simulink model "basicModel"  (R2017b)
settings: Solver=ode3  StartTime=0.0  StopTime=30  FixedStep=0.01  RelTol=1e-3  EnableMultiTasking=on
InitFcn:
  | clear;
  | clc;
  | Iniparameters
StopFcn:
  | simplot
values from neighbouring files (symbols this model uses):
  aaa = inv([kf kf kf kf ... (first row only)    [copterpara.m]
  g = 9.8    [copterpara.m]
  Ixx = 19.688e-3    (= 0.019688)    [copterpara.m]
  Iyy = 19.688e-3    (= 0.019688)    [copterpara.m]
  Izz = 3.938e-2    (= 0.03938)    [copterpara.m]
  kdphi = 8    [controlpara.m]
  kdpsai = 40    [controlpara.m]
  kdtheta = kdphi    (= 8)    [controlpara.m]
  kdx = 0.55    [controlpara.m]
  kdy = 2.0    (= 2)    [controlpara.m]
  kdz = 2.4    [controlpara.m]
  kf = 3.13e-5    (= 3.13e-05)    [copterpara.m]
  kipsai = 10    [controlpara.m]
  Kis = 0.00    (= 0)    [Iniparameters.m]
  kix = 0.001    [controlpara.m]
  kiy = 0.001    [controlpara.m]
  kiz = 0.001    [controlpara.m]
  km = 7.5e-7    (= 7.5e-07)    [copterpara.m]
  kpphi = 25    [controlpara.m]
  kppsai = 20    [controlpara.m]
  Kps = 20    [Iniparameters.m]
  kptheta = kpphi    (= 25)    [controlpara.m]
  kpx = 0.75    [controlpara.m]
  kpy = 1.4    [controlpara.m]
  kpz = 2.9    [controlpara.m]
  L = 0.25    [copterpara.m]
  m = 0.75    [copterpara.m]
  xf = 0    [controlpara.m]
  yaw = 0    [copterpara.m]
  yf = 0    [controlpara.m]
  zf = 5    [controlpara.m]
libraries: aerolibconvert2 x19, aerolibutil x7, sharedtransform x3, dspfdesign x1, sharedutil x1, aerolibnav x1
settings Model: Creator=KingBoy  LastModifiedBy=KingBoy
settings DataIOCC: LimitDataPoints=on  SaveFormat=Array
settings OptimizationCC: LifeSpan=inf
settings DebuggingCC: UnderspecifiedInitializationDetection=Classic  MergeDetectMultiDrivingBlocksExec=none  SolverPrmCheckMsg=warning  AllowSymbolicDim=off  SFUnexpectedBacktrackingDiag=warning  SFNoUnconditionalDefaultTransitionDiag=warning  SFExecutionAtInitializationDiag=none
settings HardwareCC: ProdBitPerPointer=32  ProdBitPerSizeT=32  ProdBitPerPtrDiffT=32  ProdLargestAtomicFloat=None  ProdIntDivRoundTo=Undefined  ProdEndianess=Unspecified  ProdWordSize=32  ProdHWDeviceType=32-bit Generic
settings ModelReferenceCC: PropagateSignalLabelsOutOfModel=off
settings CodeAppCC: StateflowObjectComments=on
settings GRTTargetCC: TargetLangStandard=C89/C90 (ANSI)  GeneratePreprocessorConditionals=Disable all
settings ConfigComp: CovMetricSettings=dw  CovHtmlReporting=on  CovSaveCumulativeToWorkspaceVar=on  CovSaveSingleToWorkspaceVar=on  CovExternalEMLEnable=off  CovSFcnEnable=off

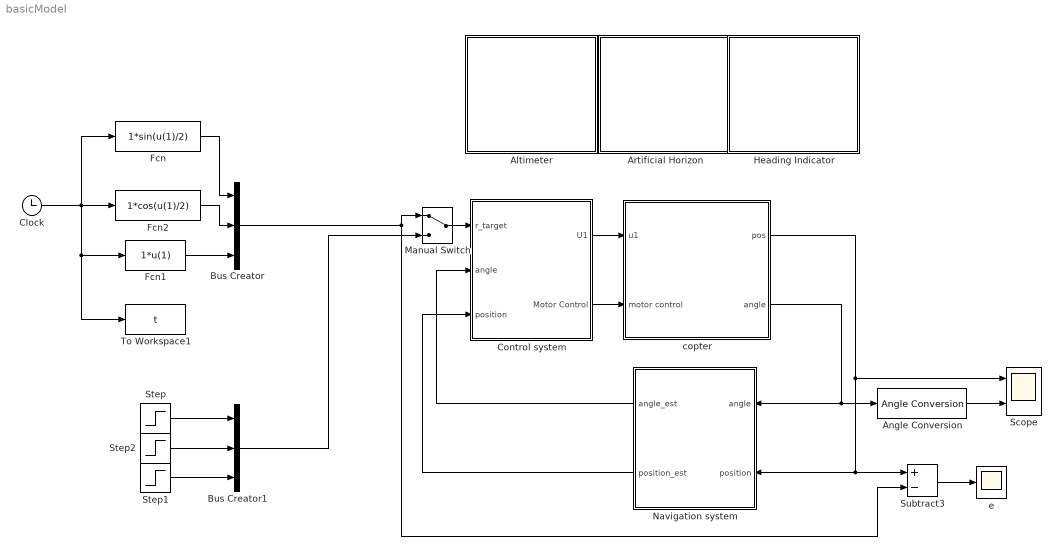
== system basicModel ==
  Altimeter : Subsystem  DialogController=aeroblksHMICreateDDGDialog  IsWebBlock=on  mask(MWDashboardBlock){webBlockId=0f36f96d-2aae-4714-b8ea-94d9972957ff, webBlockType=altimeter, ShowInLibBrowser=on, ShowInitialText=on, HMISrcModelName=basicModel}
      mask prompts: webBlockId "WebBlock Id"; webBlockType "WebBlock Type"; HMISrcModelName "Source Model"
      mask help: aeroblksHMI:aeroblkhmi:AltimeterDialogDesc
      mask Help: eval('asbhmihelp(''altimeter'')');
      mask Display:
      | if strcmp(get_param(bdroot(gcb),'BlockDiagramType'), 'library')
      |  image([(matlabroot) '/toolbox/aeroblks/aeroblks/hmi/icons/AltimeterIcon.svg'])
      | end
  Angle Conversion : aerolibconvert2/Angle Conversion  IU=rad  OU=deg
  Artificial Horizon : Subsystem  DialogController=aeroblksHMICreateDDGDialog  IsWebBlock=on  mask(MWDashboardBlock){webBlockId=fe52ae29-8116-408a-bf44-916d05edf52b, webBlockType=artificialhorizon, ShowInLibBrowser=on, ShowInitialText=on, HMISrcModelName=basicModel}
      mask prompts: webBlockId "WebBlock Id"; webBlockType "WebBlock Type"; HMISrcModelName "Source Model"
      mask help: aeroblksHMI:aeroblkhmi:ArtificialHorizonDialogDesc
      mask Help: eval('asbhmihelp(''artificialhorizon'')');
      mask Display:
      | if strcmp(get_param(bdroot(gcb),'BlockDiagramType'), 'library')
      |  image([(matlabroot) '/toolbox/aeroblks/aeroblks/hmi/icons/ArtificialHorizonIcon.svg'])
      | end
  Bus Creator : BusCreator  Inputs=3
  Bus Creator1 : BusCreator  Inputs=3
  Clock : Clock
  Control system : Subsystem
  Fcn : Fcn  Expr=1*sin(u(1)/2)
  Fcn1 : Fcn  Expr=1*u(1)
  Fcn2 : Fcn  Expr=1*cos(u(1)/2)
  Heading Indicator : Subsystem  DialogController=aeroblksHMICreateDDGDialog  IsWebBlock=on  mask(MWDashboardBlock){webBlockId=cbbc731a-5116-4125-a70b-a05ae3f6ae8f, webBlockType=headingindicator, ShowInLibBrowser=on, ShowInitialText=on, HMISrcModelName=basicModel}
      mask prompts: webBlockId "WebBlock Id"; webBlockType "WebBlock Type"; HMISrcModelName "Source Model"
      mask help: aeroblksHMI:aeroblkhmi:HeadingIndicatorDialogDesc
      mask Help: eval('asbhmihelp(''headingindicator'')');
      mask Display:
      | if strcmp(get_param(bdroot(gcb),'BlockDiagramType'), 'library')
      |  image([(matlabroot) '/toolbox/aeroblks/aeroblks/hmi/icons/HeadingIndicatorIcon.svg'])
      | end
  Manual Switch : ManualSwitch
  Navigation system : Subsystem
  Scope : Scope  NumInputPorts=2
  Step : Step  Time=0  After=xf  SampleTime=0
  Step1 : Step  Time=0  After=zf  SampleTime=0
  Step2 : Step  Time=0  After=yf  SampleTime=0
  Subtract3 : Sum  Inputs=+-
  To Workspace1 : ToWorkspace  VariableName=t  SampleTime=-1
      settings: Save2DSignal=2-D array (concatenate along first dimension)
  copter : Subsystem
  e : Scope
  wires:
  Angle Conversion/1 -> Scope/2
  Clock/1 -> To Workspace1/1, Fcn1/1, Fcn/1, Fcn2/1
  Fcn/1 -> Bus Creator/1
  Fcn2/1 -> Bus Creator/2
  Fcn1/1 -> Bus Creator/3
  Subtract3/1 -> e/1
  Bus Creator/1 -> Manual Switch/1, Subtract3/2
  copter/2(angle) -> Angle Conversion/1, Navigation system/1(angle)
  copter/1(pos) -> Scope/1, Subtract3/1, Navigation system/2(position)
  Control system/1(U1) -> copter/1(u1)
  Control system/2(Motor Control) -> copter/2(motor control)
  Navigation system/1(angle_est) -> Control system/2(angle)
  Navigation system/2(position_est) -> Control system/3(position)
  Manual Switch/1 -> Control system/1(r_target)
  Bus Creator1/1 -> Manual Switch/2
  Step/1 -> Bus Creator1/1
  Step1/1 -> Bus Creator1/3
  Step2/1 -> Bus Creator1/2

== system basicModel/Altimeter ==

== system basicModel/Artificial Horizon ==

== system basicModel/Control system ==
  r_target : Inport
  angle : Inport  Port=2
  position : Inport  Port=3
  Attitude Control : Subsystem
  PositionControl : Subsystem
  U1 : Outport
  Motor Control : Outport  Port=2
  wires:
  PositionControl/2(angle_des) -> Attitude Control/1(angle_des)
  angle/1 -> Attitude Control/2(angle_est)
  PositionControl/1(u1) -> U1/1
  Attitude Control/1(motor control) -> Motor Control/1
  position/1 -> PositionControl/2(r_pos)
  r_target/1 -> PositionControl/1(r_target)

== system basicModel/Heading Indicator ==

== system basicModel/Navigation system ==
  angle : Inport
  position : Inport  Port=2
  Attitude estimate : Subsystem
  gps sensor : Subsystem
  inertial sensor : Subsystem
  position estimate : Subsystem
  angle_est : Outport
  position_est : Outport  Port=2
  wires:
  position/1 -> gps sensor/1(pos)
  angle/1 -> inertial sensor/1(angle)
  gps sensor/1(GPSpos) -> position estimate/1(GPSpos)
  position estimate/1(postion_est) -> position_est/1
  inertial sensor/1(acc gyro mag) -> Attitude estimate/1(acc gyro mag)
  Attitude estimate/1(angle_est) -> angle_est/1
  inertial sensor/2(acc gyro mag1) -> Attitude estimate/2(acc gyro mag1)

== system basicModel/copter ==
  u1 : Inport
  motor control : Inport  Port=2
  Moter Dynamic : Subsystem
  Rigid Body Dynamic : Subsystem
  pos : Outport
  angle : Outport  Port=2
  wires:
  u1/1 -> Moter Dynamic/1(u1)
  Rigid Body Dynamic/2(angle) -> angle/1
  motor control/1 -> Moter Dynamic/2(d_wphi)
  Rigid Body Dynamic/1(xyzt) -> pos/1
  Moter Dynamic/2(M) -> Rigid Body Dynamic/2(M)
  Moter Dynamic/1(T) -> Rigid Body Dynamic/1(T)

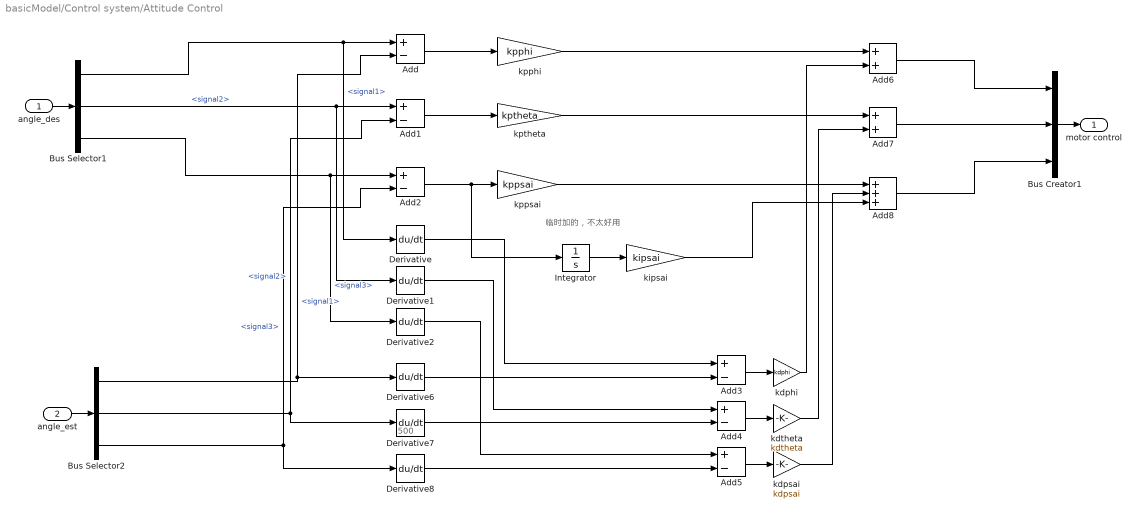
== system basicModel/Control system/Attitude Control ==
  note: 临时加的，不太好用
  note: 500
  angle_des : Inport
  angle_est : Inport  Port=2
  Add{,1..5} (6 alike) : Sum  Inputs=+-
  Add6 : Sum
  Add7 : Sum
  Add8 : Sum  Inputs=+++
  Bus Creator1 : BusCreator  Inputs=3
  Bus Selector1 : BusSelector  OutputSignals=signal1,signal2,signal3
  Bus Selector2 : BusSelector  OutputSignals=signal1,signal2,signal3
  Derivative{,1..2,6..8} (6 alike) : Derivative  CoefficientInTFapproximation=500
  Integrator : Integrator
  kdphi : Gain  Gain=kdphi
  kdpsai : Gain  Gain=kdpsai
  kdtheta : Gain  Gain=kdtheta
  kipsai : Gain  Gain=kipsai
  kpphi : Gain  Gain=kpphi
  kppsai : Gain  Gain=kppsai
  kptheta : Gain  Gain=kptheta
  motor control : Outport
  wires:
  Bus Selector1/1 -> Add/1, Derivative/1  "<signal1>"
  Bus Selector2/1 -> Add/2, Derivative6/1  "<signal1>"
  Add/1 -> kpphi/1
  Bus Selector1/2 -> Derivative1/1, Add1/1  "<signal2>"
  Bus Selector2/2 -> Add1/2, Derivative7/1  "<signal2>"
  Add1/1 -> kptheta/1
  Add2/1 -> Integrator/1, kppsai/1
  Bus Selector1/3 -> Derivative2/1, Add2/1  "<signal3>"
  Bus Selector2/3 -> Add2/2, Derivative8/1  "<signal3>"
  Add3/1 -> kdphi/1
  Add4/1 -> kdtheta/1
  Add5/1 -> kdpsai/1
  kpphi/1 -> Add6/1
  kdphi/1 -> Add6/2
  kptheta/1 -> Add7/1
  kdtheta/1 -> Add7/2
  kppsai/1 -> Add8/1
  kdpsai/1 -> Add8/2
  Derivative/1 -> Add3/1
  Derivative1/1 -> Add4/1
  Derivative2/1 -> Add5/1
  Derivative6/1 -> Add3/2
  Derivative7/1 -> Add4/2
  Derivative8/1 -> Add5/2
  angle_est/1 -> Bus Selector2/1
  angle_des/1 -> Bus Selector1/1
  Bus Creator1/1 -> motor control/1
  Add6/1 -> Bus Creator1/1
  Add7/1 -> Bus Creator1/2
  Add8/1 -> Bus Creator1/3
  Integrator/1 -> kipsai/1
  kipsai/1 -> Add8/3

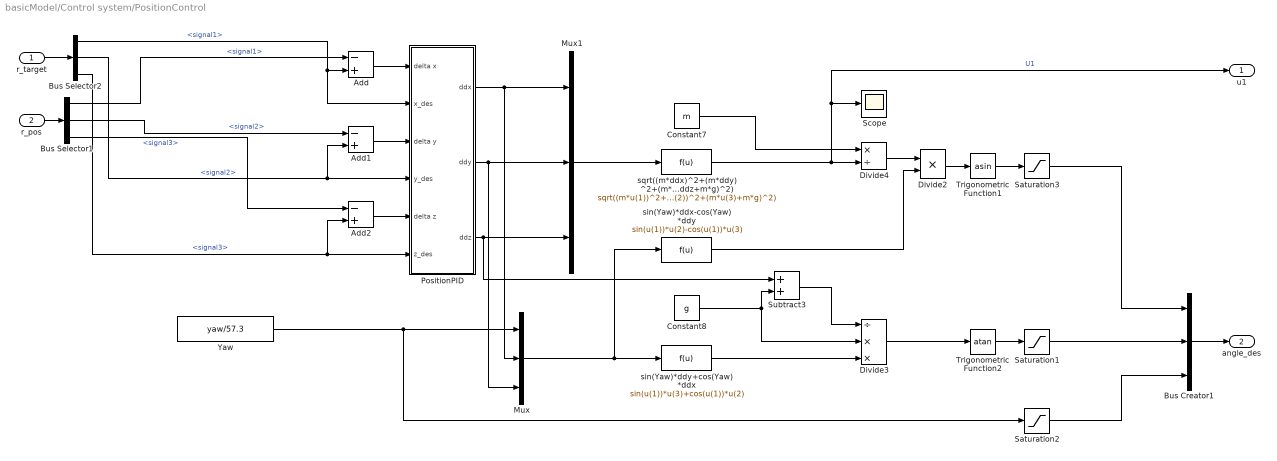
== system basicModel/Control system/PositionControl ==
  r_target : Inport
  r_pos : Inport  Port=2
  Add : Sum  Inputs=-+
  Add1 : Sum  Inputs=-+
  Add2 : Sum  Inputs=-+
  Bus Creator1 : BusCreator  Inputs=3
  Bus Selector1 : BusSelector  OutputSignals=signal1,signal2,signal3
  Bus Selector2 : BusSelector  OutputSignals=signal1,signal2,signal3
  Constant7 : Constant  Value=m
  Constant8 : Constant  Value=g
  Divide2 : Product  Inputs=**
  Divide3 : Product  Inputs=/**
  Divide4 : Product  Inputs=*/
  Mux : Mux  Inputs=3
  Mux1 : Mux  Inputs=3
  PositionPID : Subsystem
  Saturation1 : Saturate  UpperLimit=90/57.3  LowerLimit=-90/57.3
  Saturation2 : Saturate  UpperLimit=90/57.3  LowerLimit=-90/57.3
  Saturation3 : Saturate  UpperLimit=90/57.3  LowerLimit=-90/57.3
  Scope : Scope
  Subtract3 : Sum
  Trigonometric Function1 : Trigonometry  Operator=asin
  Trigonometric Function2 : Trigonometry  Operator=atan
  Yaw : Constant  Value=yaw/57.3
  sin(Yaw)*ddx-cos(Yaw)*ddy : Fcn  Expr=sin(u(1))*u(2)-cos(u(1))*u(3)
  sin(Yaw)*ddy+cos(Yaw)*ddx : Fcn  Expr=sin(u(1))*u(3)+cos(u(1))*u(2)
  sqrt((m*ddx)^2+(m*ddy)^2+(m*ddz+m*g)^2) : Fcn  Expr=sqrt((m*u(1))^2+(m*u(2))^2+(m*u(3)+m*g)^2)
  u1 : Outport
  angle_des : Outport  Port=2
  wires:
  Bus Selector1/1 -> Add/1  "<signal1>"
  Add/1 -> PositionPID/1(delta x)
  Bus Selector1/2 -> Add1/1  "<signal2>"
  Bus Selector2/2 -> Add1/2, PositionPID/4(y_des)  "<signal2>"
  Add1/1 -> PositionPID/3(delta y)
  Bus Selector1/3 -> Add2/1  "<signal3>"
  Bus Selector2/3 -> Add2/2, PositionPID/6(z_des)  "<signal3>"
  Add2/1 -> PositionPID/5(delta z)
  PositionPID/2(ddy) -> Mux/3, Mux1/2
  sqrt((m*ddx)^2+(m*ddy)^2+(m*ddz+m*g)^2)/1 -> u1/1, Scope/1, Divide4/2  "U1"
  PositionPID/3(ddz) -> Subtract3/1, Mux1/3
  sin(Yaw)*ddx-cos(Yaw)*ddy/1 -> Divide2/2
  Divide3/1 -> Trigonometric Function2/1
  Constant7/1 -> Divide4/1
  Divide4/1 -> Divide2/1
  Constant8/1 -> Divide3/2, Subtract3/2
  Trigonometric Function2/1 -> Saturation1/1
  Trigonometric Function1/1 -> Saturation3/1
  Divide2/1 -> Trigonometric Function1/1
  PositionPID/1(ddx) -> Mux1/1, Mux/2
  Yaw/1 -> Mux/1, Saturation2/1
  Subtract3/1 -> Divide3/1
  Saturation3/1 -> Bus Creator1/1
  Saturation1/1 -> Bus Creator1/2
  Saturation2/1 -> Bus Creator1/3
  Mux/1 -> sin(Yaw)*ddx-cos(Yaw)*ddy/1, sin(Yaw)*ddy+cos(Yaw)*ddx/1
  Mux1/1 -> sqrt((m*ddx)^2+(m*ddy)^2+(m*ddz+m*g)^2)/1
  sin(Yaw)*ddy+cos(Yaw)*ddx/1 -> Divide3/3
  r_pos/1 -> Bus Selector1/1
  r_target/1 -> Bus Selector2/1
  Bus Selector2/1 -> PositionPID/2(x_des), Add/2  "<signal1>"
  Bus Creator1/1 -> angle_des/1

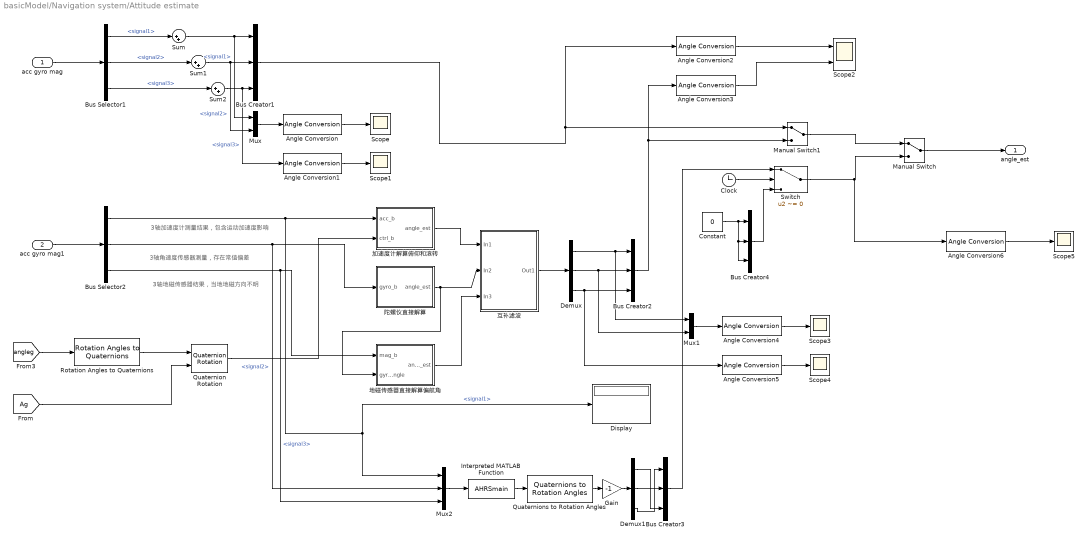
== system basicModel/Navigation system/Attitude estimate ==
  note: 3轴加速度计测量结果，包含运动加速度影响
  note: 3轴角速度传感器测量，存在常值偏差
  note: 3轴地磁传感器结果，当地地磁方向不明
  acc gyro mag : Inport
  acc gyro mag1 : Inport  Port=2
  Angle Conversion{,1..6} (7 alike) : aerolibconvert2/Angle Conversion  IU=rad  OU=deg
  Bus Creator{1..4} (4 alike) : BusCreator  Inputs=3
  Bus Selector1 : BusSelector  OutputSignals=signal1,signal2,signal3
  Bus Selector2 : BusSelector  OutputSignals=signal1,signal2,signal3
  Clock : Clock
  Constant : Constant  Value=0
  Demux : Demux  Outputs=3
  Demux1 : Demux  Outputs=3
  Display : Display
  Gain : Gain  Gain=-1
  Interpreted MATLAB Function : MATLABFcn  MATLABFcn=AHRSmain
  Manual Switch : ManualSwitch
  Manual Switch1 : ManualSwitch
  Mux : Mux  Inputs=2
  Mux1 : Mux  Inputs=2
  Mux2 : Mux  Inputs=3
  Quaternion Rotation : aerolibutil/Quaternion Rotation
  Quaternions to Rotation Angles : sharedtransform/Quaternions to Rotation Angles  rotationOrder=ZYX
      settings: SourceProductBaseCode=AE
  Rotation Angles to Quaternions : sharedtransform/Rotation Angles to Quaternions  rotationOrder=ZYX
      settings: SourceProductName=Aerospace Blockset  SourceProductBaseCode=AE
  Scope{,1,3..5} (5 alike) : Scope
  Scope2 : Scope  NumInputPorts=2
  Sum : Sum  Inputs=|++
  Sum1 : Sum  Inputs=|++
  Sum2 : Sum  Inputs=|++
  Switch : Switch  Criteria=u2 ~= 0
  互补滤波 : Subsystem
  加速度计解算俯仰和滚转 : Subsystem
  地磁传感器直接解算偏航角 : Subsystem
  陀螺仪直接解算 : Subsystem
  angle_est : Outport
  wires:
  acc gyro mag/1 -> Bus Selector1/1
  Bus Creator1/1 -> Manual Switch1/1, Angle Conversion2/1
  Bus Selector1/1 -> Sum/1  "<signal1>"
  Bus Selector1/2 -> Sum1/1  "<signal2>"
  Bus Selector1/3 -> Sum2/1  "<signal3>"
  Sum/1 -> Mux/1, Bus Creator1/1  "<signal1>"
  Sum1/1 -> Mux/2, Bus Creator1/2  "<signal2>"
  Sum2/1 -> Angle Conversion1/1, Bus Creator1/3  "<signal3>"
  Mux/1 -> Angle Conversion/1
  Angle Conversion/1 -> Scope/1
  Angle Conversion1/1 -> Scope1/1
  acc gyro mag1/1 -> Bus Selector2/1
  Bus Selector2/3 -> Mux2/3, 地磁传感器直接解算偏航角/1(mag_b)  "<signal3>"
  Bus Selector2/2 -> Mux2/2, 陀螺仪直接解算/1(gyro_b)  "<signal2>"
  Rotation Angles to Quaternions/1 -> Quaternion Rotation/1
  [angleg] -> Rotation Angles to Quaternions/1
  [Ag] -> Quaternion Rotation/2
  Bus Selector2/1 -> Display/1, Mux2/1, 加速度计解算俯仰和滚转/1(acc_b)  "<signal1>"
  Quaternion Rotation/1 -> 加速度计解算俯仰和滚转/2(ctrl_b)
  加速度计解算俯仰和滚转/1(angle_est) -> 互补滤波/1(In1)
  陀螺仪直接解算/1(angle_est) -> 地磁传感器直接解算偏航角/2(gyro angle), 互补滤波/2(In2)
  互补滤波/1(Out1) -> Demux/1
  Demux/1 -> Mux1/1, Bus Creator2/1
  Demux/2 -> Mux1/2, Bus Creator2/2
  地磁传感器直接解算偏航角/1(angle_est) -> 互补滤波/3(In3)
  Bus Creator2/1 -> Manual Switch1/2, Angle Conversion3/1
  Manual Switch/1 -> angle_est/1
  Angle Conversion2/1 -> Scope2/1
  Angle Conversion3/1 -> Scope2/2
  Demux/3 -> Angle Conversion5/1, Bus Creator2/3
  Angle Conversion4/1 -> Scope3/1
  Angle Conversion5/1 -> Scope4/1
  Mux1/1 -> Angle Conversion4/1
  Mux2/1 -> Interpreted MATLAB Function/1
  Interpreted MATLAB Function/1 -> Quaternions to Rotation Angles/1
  Quaternions to Rotation Angles/1 -> Gain/1
  Angle Conversion6/1 -> Scope5/1
  Demux1/1 -> Bus Creator3/3
  Demux1/2 -> Bus Creator3/2
  Demux1/3 -> Bus Creator3/1
  Bus Creator3/1 -> Switch/1
  Gain/1 -> Demux1/1
  Clock/1 -> Switch/2
  Switch/1 -> Angle Conversion6/1, Manual Switch/2
  Constant/1 -> Bus Creator4/3, Bus Creator4/2, Bus Creator4/1
  Bus Creator4/1 -> Switch/3
  Manual Switch1/1 -> Manual Switch/1

== system basicModel/Navigation system/gps sensor ==
  pos : Inport
  Bus Creator1 : BusCreator  Inputs=3
  Bus Selector1 : BusSelector  OutputSignals=signal1,signal2,signal3
  Manual Switch : ManualSwitch  CurrentSetting=0
  Random Number : RandomNumber  Variance=100  Seed=10  SampleTime=0.01
  Random Number1 : RandomNumber  Variance=100  Seed=11  SampleTime=0.01
  Random Number2 : RandomNumber  Variance=100  Seed=12  SampleTime=0.01
  Scope : Scope
  Sum : Sum  Inputs=|++
  Sum1 : Sum  Inputs=|++
  Sum2 : Sum  Inputs=|++
  GPSpos : Outport
  wires:
  pos/1 -> Manual Switch/2, Bus Selector1/1
  Bus Creator1/1 -> Manual Switch/1
  Bus Selector1/1 -> Sum/1  "<signal1>"
  Bus Selector1/2 -> Sum1/1  "<signal2>"
  Bus Selector1/3 -> Sum2/1  "<signal3>"
  Random Number/1 -> Sum/2
  Sum/1 -> Bus Creator1/1
  Manual Switch/1 -> Scope/1, GPSpos/1
  Sum2/1 -> Bus Creator1/3
  Sum1/1 -> Bus Creator1/2
  Random Number1/1 -> Sum1/2
  Random Number2/1 -> Sum2/2

== system basicModel/Navigation system/inertial sensor ==
  angle : Inport
  9轴惯性测量单元 : Subsystem
  Bus Creator1 : BusCreator  Inputs=3
  Bus Selector1 : BusSelector  OutputSignals=signal1,signal2,signal3
  acc gyro mag : Outport
  acc gyro mag1 : Outport  Port=2
  wires:
  angle/1 -> Bus Selector1/1
  Bus Creator1/1 -> acc gyro mag/1
  Bus Selector1/1 -> Bus Creator1/1  "<signal1>"
  Bus Selector1/2 -> Bus Creator1/2  "<signal2>"
  Bus Selector1/3 -> Bus Creator1/3  "<signal3>"
  9轴惯性测量单元/1(acc gyro mag) -> acc gyro mag1/1

== system basicModel/Navigation system/position estimate ==
  GPSpos : Inport
  Bus Creator1 : BusCreator  Inputs=3
  Bus Selector1 : BusSelector  OutputSignals=signal1,signal2,signal3
  Scope : Scope
  postion_est : Outport
  wires:
  GPSpos/1 -> Bus Selector1/1
  Bus Creator1/1 -> Scope/1, postion_est/1
  Bus Selector1/1 -> Bus Creator1/1  "<signal1>"
  Bus Selector1/2 -> Bus Creator1/2  "<signal2>"
  Bus Selector1/3 -> Bus Creator1/3  "<signal3>"

== system basicModel/copter/Moter Dynamic ==
  note: 电机惯性延迟50ms
  u1 : Inport
  d_wphi : Inport  Port=2
  Bus Selector1 : BusSelector  OutputSignals=signal1,signal2,signal3
  Gain : Gain  Gain=kf
  Gain1 : Gain  Gain=20
  Gain4 : Gain  Gain=km
  Integrator : Integrator
  Mux : Mux
  Scope : Scope  NumInputPorts=2
  Scope1 : Scope
  Scope2 : Scope
  Sum : Sum  Inputs=+-
  w : Subsystem
  T : Outport
  M : Outport  Port=2
  wires:
  u1/1 -> w/1(u1)
  w/4(w4_des) -> Mux/4
  w/3(w3_des) -> Mux/3
  w/1(w1_des) -> Mux/1
  w/2(w2_des) -> Mux/2
  Gain4/1 -> M/1
  Mux/1 -> Scope/1, Sum/1
  d_wphi/1 -> Scope2/1, Bus Selector1/1
  Bus Selector1/1 -> w/2(ddphi)  "<signal1>"
  Bus Selector1/2 -> w/3(ddtheta)  "<signal2>"
  Bus Selector1/3 -> w/4(ddpsi)  "<signal3>"
  Integrator/1 -> Scope/2, Gain4/1, Scope1/1, Gain/1, Sum/2
  Sum/1 -> Gain1/1
  Gain1/1 -> Integrator/1
  Gain/1 -> T/1

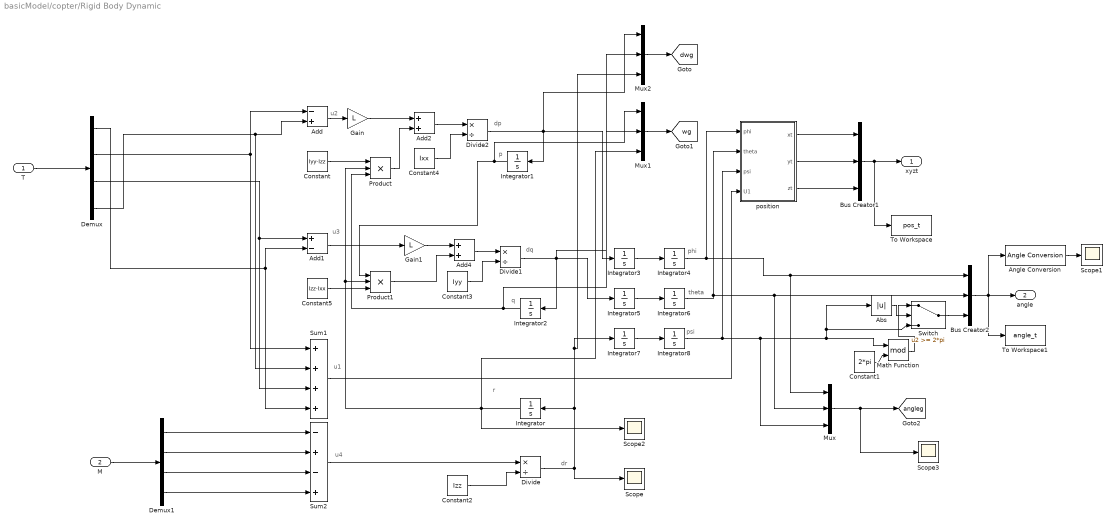
== system basicModel/copter/Rigid Body Dynamic ==
  note: psi
  note: theta
  note: phi
  note: p
  note: q
  note: dq
  note: dp
  note: u4
  note: u3
  note: u2
  note: u1
  note: r
  note: dr
  T : Inport
  M : Inport  Port=2
  Abs : Abs
  Add : Sum  Inputs=-+
  Add1 : Sum  Inputs=+-
  Add2 : Sum
  Add4 : Sum
  Angle Conversion : aerolibconvert2/Angle Conversion  IU=rad  OU=deg
  Bus Creator1 : BusCreator  Inputs=3
  Bus Creator2 : BusCreator  Inputs=3
  Constant : Constant  Value=Iyy-Izz
  Constant1 : Constant  Value=2*pi
  Constant2 : Constant  Value=Izz
  Constant3 : Constant  Value=Iyy
  Constant4 : Constant  Value=Ixx
  Constant5 : Constant  Value=Izz-Ixx
  Demux : Demux
  Demux1 : Demux
  Divide : Product  Inputs=*/
  Divide1 : Product  Inputs=*/
  Divide2 : Product  Inputs=*/
  Gain : Gain  Gain=L
  Gain1 : Gain  Gain=L
  Integrator : Integrator  UpperSaturationLimit=50  LowerSaturationLimit=-50
  Integrator{1..8} (8 alike) : Integrator
  Math Function : Math  Operator=mod  SaturateOnIntegerOverflow=on
  Mux : Mux  Inputs=3
  Mux1 : Mux  Inputs=3
  Mux2 : Mux  Inputs=3
  Product : Product  Inputs=3
  Product1 : Product  Inputs=3
  Scope{,1..3} (4 alike) : Scope
  Sum1 : Sum  Inputs=++++
  Sum2 : Sum  Inputs=-+-+
  Switch : Switch  Threshold=2*pi
  To Workspace : ToWorkspace  VariableName=pos_t  SampleTime=-1
      settings: Save2DSignal=2-D array (concatenate along first dimension)
  To Workspace1 : ToWorkspace  VariableName=angle_t  SampleTime=-1
      settings: Save2DSignal=2-D array (concatenate along first dimension)
  position : Subsystem
  xyzt : Outport
  angle : Outport  Port=2
  tag scope: angleg=global, dwg=global, wg=global
  wires:
  Demux/2 -> Add/1, Sum1/1
  Demux/4 -> Add/2, Sum1/2
  Add/1 -> Gain/1
  Add1/1 -> Gain1/1
  Gain/1 -> Add2/1
  Constant/1 -> Product/1
  Product/1 -> Add2/2
  Demux1/2 -> Sum2/2
  Demux1/3 -> Sum2/3
  Demux1/4 -> Sum2/4
  Constant2/1 -> Divide/2
  Integrator/1 -> Mux1/3, Product/2, Product1/2, Scope2/1
  Gain1/1 -> Add4/1
  Demux/3 -> Add1/1, Sum1/3
  Demux/1 -> Add1/2, Sum1/4
  Add4/1 -> Divide1/1
  Constant3/1 -> Divide1/2
  Sum1/1 -> position/4(U1)
  Add2/1 -> Divide2/1
  Constant4/1 -> Divide2/2
  Integrator2/1 -> Mux1/2, Product/3
  Constant5/1 -> Product1/3
  Product1/1 -> Add4/2
  Integrator1/1 -> Mux1/1, Product1/1
  Integrator4/1 -> Bus Creator2/1, Mux/1, position/1(phi)
  Bus Creator2/1 -> Angle Conversion/1, To Workspace1/1, angle/1
  position/1(xt) -> Bus Creator1/1
  position/2(yt) -> Bus Creator1/2
  position/3(zt) -> Bus Creator1/3
  Integrator3/1 -> Integrator4/1
  Integrator5/1 -> Integrator6/1
  Integrator7/1 -> Integrator8/1
  Sum2/1 -> Divide/1
  Bus Creator1/1 -> To Workspace/1, xyzt/1
  T/1 -> Demux/1
  Demux1/1 -> Sum2/1
  M/1 -> Demux1/1
  Mux1/1 -> [wg]
  Divide/1 -> Scope/1, Mux2/3, Integrator7/1, Integrator/1
  Divide1/1 -> Mux2/2, Integrator5/1, Integrator2/1
  Divide2/1 -> Mux2/1, Integrator1/1, Integrator3/1
  Integrator6/1 -> Bus Creator2/2, Mux/2, position/2(theta)
  Mux/1 -> Scope3/1, [angleg]
  Mux2/1 -> [dwg]
  Constant1/1 -> Math Function/2
  Switch/1 -> Bus Creator2/3
  Integrator8/1 -> position/3(psi), Math Function/1, Abs/1, Switch/3, Mux/3
  Math Function/1 -> Switch/1
  Abs/1 -> Switch/2
  Angle Conversion/1 -> Scope1/1

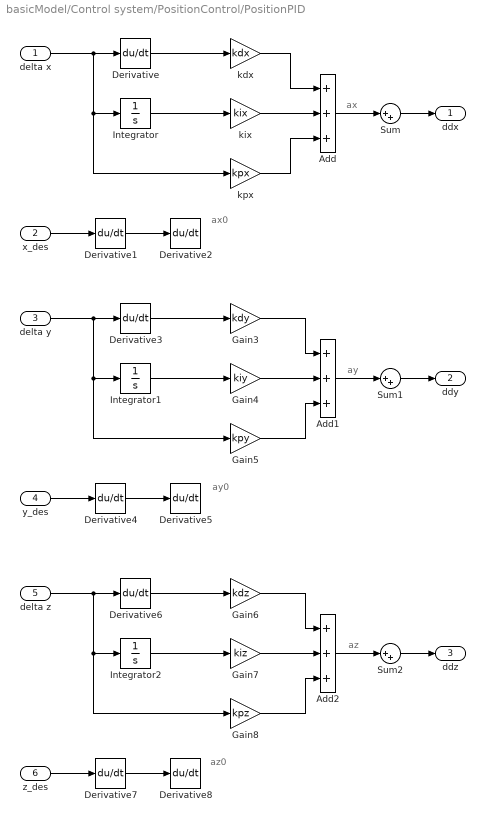
== system basicModel/Control system/PositionControl/PositionPID ==
  note: az
  note: ay
  note: ax
  note: az0
  note: ay0
  note: ax0
  delta x : Inport
  x_des : Inport  Port=2
  delta y : Inport  Port=3
  y_des : Inport  Port=4
  delta z : Inport  Port=5
  z_des : Inport  Port=6
  Add : Sum  Inputs=+++
  Add1 : Sum  Inputs=+++
  Add2 : Sum  Inputs=+++
  Derivative{,1..5,7..8} (8 alike) : Derivative  CoefficientInTFapproximation=500
  Derivative6 : Derivative
  Gain3 : Gain  Gain=kdy
  Gain4 : Gain  Gain=kiy
  Gain5 : Gain  Gain=kpy
  Gain6 : Gain  Gain=kdz
  Gain7 : Gain  Gain=kiz
  Gain8 : Gain  Gain=kpz
  Integrator : Integrator
  Integrator1 : Integrator
  Integrator2 : Integrator
  Sum : Sum  Inputs=|++
  Sum1 : Sum  Inputs=|++
  Sum2 : Sum  Inputs=|++
  kdx : Gain  Gain=kdx
  kix : Gain  Gain=kix
  kpx : Gain  Gain=kpx
  ddx : Outport
  ddy : Outport  Port=2
  ddz : Outport  Port=3
  wires:
  delta x/1 -> kpx/1, Integrator/1, Derivative/1
  Derivative/1 -> kdx/1
  kdx/1 -> Add/1
  Integrator/1 -> kix/1
  kix/1 -> Add/2
  kpx/1 -> Add/3
  Add/1 -> Sum/1
  Derivative1/1 -> Derivative2/1
  x_des/1 -> Derivative1/1
  Sum/1 -> ddx/1
  delta y/1 -> Gain5/1, Integrator1/1, Derivative3/1
  Derivative3/1 -> Gain3/1
  Gain3/1 -> Add1/1
  Integrator1/1 -> Gain4/1
  Gain4/1 -> Add1/2
  Gain5/1 -> Add1/3
  Add1/1 -> Sum1/1
  Derivative4/1 -> Derivative5/1
  y_des/1 -> Derivative4/1
  Sum1/1 -> ddy/1
  delta z/1 -> Gain8/1, Integrator2/1, Derivative6/1
  Derivative6/1 -> Gain6/1
  Gain6/1 -> Add2/1
  Integrator2/1 -> Gain7/1
  Gain7/1 -> Add2/2
  Gain8/1 -> Add2/3
  Add2/1 -> Sum2/1
  Derivative7/1 -> Derivative8/1
  z_des/1 -> Derivative7/1
  Sum2/1 -> ddz/1

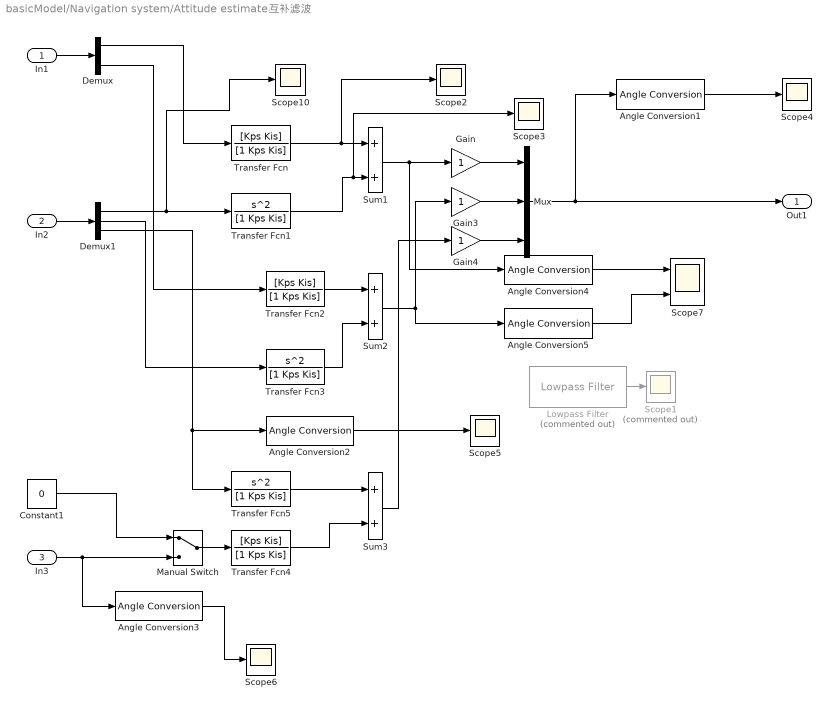
== system basicModel/Navigation system/Attitude estimate/互补滤波 ==
  In1 : Inport
  In2 : Inport  Port=2
  In3 : Inport  Port=3
  Angle Conversion{1..5} (5 alike) : aerolibconvert2/Angle Conversion  IU=rad  OU=deg
  Constant1 : Constant  Value=0
  Demux : Demux  Outputs=2
  Demux1 : Demux  Outputs=3
  Gain : Gain  OutMin=-pi/2  OutMax=pi/2
  Gain3 : Gain  OutMin=-pi/2  OutMax=pi/2
  Gain4 : Gain  OutMin=-pi/2  OutMax=pi/2
  Lowpass Filter : dspfdesign/Lowpass Filter  Commented=on  FilterType=FIR  DesignForMinimumOrder=on  FilterOrder=50  PassbandFrequency=4e1  StopbandFrequency=10e1  PassbandRipple=0.1  StopbandAttenuation=80  InheritSampleRate=on  SampleRate=44100  SimulateUsing=Interpreted execution  roundingMode=Floor  coeffsDataTypeStr=fixdt(1,16)
  Manual Switch : ManualSwitch
  Mux : Mux  Inputs=3
  Scope1 : Scope  Commented=on
  Scope{2..6,10} (6 alike) : Scope
  Scope7 : Scope  NumInputPorts=2
  Sum1 : Sum
  Sum2 : Sum
  Sum3 : Sum
  Transfer Fcn : TransferFcn  Numerator=[Kps Kis]  Denominator=[1 Kps Kis]
  Transfer Fcn1 : TransferFcn  Numerator=[1 0 0]  Denominator=[1 Kps Kis]
  Transfer Fcn2 : TransferFcn  Numerator=[Kps Kis]  Denominator=[1 Kps Kis]
  Transfer Fcn3 : TransferFcn  Numerator=[1 0 0]  Denominator=[1 Kps Kis]
  Transfer Fcn4 : TransferFcn  Numerator=[Kps Kis]  Denominator=[1 Kps Kis]
  Transfer Fcn5 : TransferFcn  Numerator=[1 0 0]  Denominator=[1 Kps Kis]
  Out1 : Outport
  wires:
  Transfer Fcn1/1 -> Scope3/1, Sum1/2
  In2/1 -> Demux1/1
  In1/1 -> Demux/1
  Transfer Fcn/1 -> Scope2/1, Sum1/1
  Demux/1 -> Transfer Fcn/1
  Transfer Fcn3/1 -> Sum2/2
  Transfer Fcn2/1 -> Sum2/1
  Demux1/1 -> Scope10/1, Transfer Fcn1/1
  Demux/2 -> Transfer Fcn2/1
  Demux1/2 -> Transfer Fcn3/1
  Sum1/1 -> Gain/1, Angle Conversion4/1
  Sum2/1 -> Gain3/1, Angle Conversion5/1
  Lowpass Filter/1 -> Scope1/1
  Mux/1 -> Angle Conversion1/1, Out1/1
  Demux1/3 -> Transfer Fcn5/1, Angle Conversion2/1
  Angle Conversion1/1 -> Scope4/1
  In3/1 -> Manual Switch/2, Angle Conversion3/1
  Transfer Fcn5/1 -> Sum3/1
  Sum3/1 -> Gain4/1
  Transfer Fcn4/1 -> Sum3/2
  Angle Conversion2/1 -> Scope5/1
  Angle Conversion3/1 -> Scope6/1
  Angle Conversion4/1 -> Scope7/1
  Angle Conversion5/1 -> Scope7/2
  Gain/1 -> Mux/1
  Gain3/1 -> Mux/2
  Gain4/1 -> Mux/3
  Constant1/1 -> Manual Switch/1
  Manual Switch/1 -> Transfer Fcn4/1

== system basicModel/Navigation system/Attitude estimate/加速度计解算俯仰和滚转 ==
  acc_b : Inport
  ctrl_b : Inport  Port=2
  Angle Conversion1 : aerolibconvert2/Angle Conversion  IU=rad  OU=deg
  Constant : Constant  Value=[0 0 0]
  Data Store Memory : DataStoreMemory  ReadBeforeWriteMsg=warning  WriteAfterWriteMsg=warning  WriteAfterReadMsg=warning  InitialValue=[0;0]  ShowAdditionalParam=off
  Data Store Read : DataStoreRead
  Data Store Write : DataStoreWrite
  Gain : Gain  Gain=0.1
  Gain1 : Gain  Gain=0.9
  Manual Switch1 : ManualSwitch
  Mux : Mux  Inputs=2
  Mux1 : Mux  Inputs=2
  Scope2 : Scope
  Sum : Sum  Inputs=|++
  Sum1 : Sum  Inputs=+-
  x-fai : Fcn  Expr=asin(u(2)/9.8/cos(u(4)))
  y-theta : Fcn  Expr=asin(-u(1)/9.8)
  angle_est : Outport
  wires:
  x-fai/1 -> Mux/1
  Mux1/1 -> x-fai/1
  y-theta/1 -> Mux1/2, Mux/2
  ctrl_b/1 -> Manual Switch1/1
  acc_b/1 -> Sum1/1
  Sum1/1 -> Mux1/1, y-theta/1
  Manual Switch1/1 -> Sum1/2
  Constant/1 -> Manual Switch1/2
  Angle Conversion1/1 -> Scope2/1
  Gain1/1 -> Sum/1
  Data Store Read/1 -> Gain/1
  Gain/1 -> Sum/2
  Mux/1 -> Angle Conversion1/1, angle_est/1

== system basicModel/Navigation system/Attitude estimate/地磁传感器直接解算偏航角 ==
  note: 牛顿法求解
  note: $$f=(C11C23 - C21C13)C31Bx +(C11By - C21Bx)(C11C33 - C31C13) - C11(C11C23 - C21C13)Bz = 0$$
  mag_b : Inport
  gyro angle : Inport  Port=2
  Angle Conversion1 : aerolibconvert2/Angle Conversion  IU=rad  OU=deg
  Angle Conversion2 : aerolibconvert2/Angle Conversion  IU=rad  OU=deg
  Discrete Filter : DiscreteFilter  SampleTime=0.01
  MATLAB Function : MATLAB Function  TreatAsAtomicUnit=on
  Mux : Mux  Inputs=2
  Scope1 : Scope
  Scope2 : Scope
  angle_est : Outport
  wires:
  Angle Conversion1/1 -> Scope2/1
  mag_b/1 -> Angle Conversion1/1, Mux/2
  gyro angle/1 -> Mux/1
  Angle Conversion2/1 -> Scope1/1
  Mux/1 -> MATLAB Function/1(u)
  MATLAB Function/1(y) -> Discrete Filter/1
  Discrete Filter/1 -> Angle Conversion2/1, angle_est/1

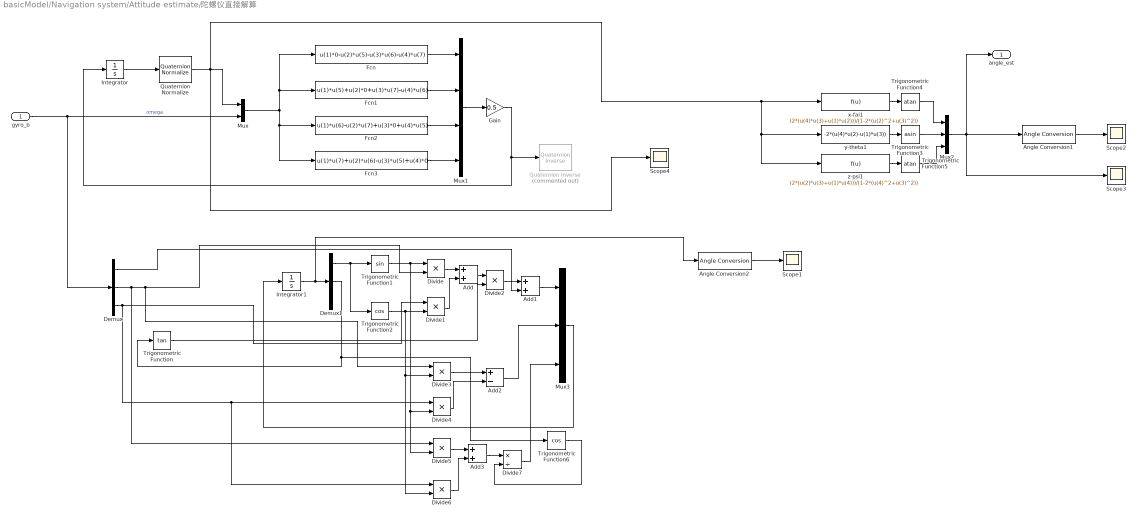
== system basicModel/Navigation system/Attitude estimate/陀螺仪直接解算 ==
  gyro_b : Inport
  Add : Sum
  Add1 : Sum
  Add2 : Sum  Inputs=+-
  Add3 : Sum
  Angle Conversion1 : aerolibconvert2/Angle Conversion  IU=rad  OU=deg
  Angle Conversion2 : aerolibconvert2/Angle Conversion  IU=rad  OU=deg
  Demux : Demux  Outputs=3
  Demux1 : Demux  Outputs=3
  Divide{,1..6} (7 alike) : Product  Inputs=**
  Divide7 : Product  Inputs=*/
  Fcn : Fcn  Expr=u(1)*0-u(2)*u(5)-u(3)*u(6)-u(4)*u(7)
  Fcn1 : Fcn  Expr=u(1)*u(5)+u(2)*0+u(3)*u(7)-u(4)*u(6)
  Fcn2 : Fcn  Expr=u(1)*u(6)-u(2)*u(7)+u(3)*0+u(4)*u(5)
  Fcn3 : Fcn  Expr=u(1)*u(7)+u(2)*u(6)-u(3)*u(5)+u(4)*0
  Gain : Gain  Gain=0.5
  Integrator : Integrator  InitialCondition=[1 0 0 0]
  Integrator1 : Integrator  InitialCondition=[0 0 0]
  Mux : Mux  Inputs=2
  Mux1 : Mux
  Mux2 : Mux  Inputs=3
  Mux3 : Mux  Inputs=3
  Quaternion Inverse : aerolibutil/Quaternion Inverse  Commented=on
      settings: SourceProductName=Aerospace Blockset
  Quaternion Normalize : sharedutil/Quaternion Normalize
      settings: SourceProductName=Aerospace Blockset  SourceProductBaseCode=AE
  Scope{1..4} (4 alike) : Scope
  Trigonometric Function : Trigonometry  Operator=tan
  Trigonometric Function1 : Trigonometry
  Trigonometric Function2 : Trigonometry  Operator=cos
  Trigonometric Function3 : Trigonometry  Operator=asin
  Trigonometric Function4 : Trigonometry  Operator=atan
  Trigonometric Function5 : Trigonometry  Operator=atan
  Trigonometric Function6 : Trigonometry  Operator=cos
  x-fai1 : Fcn  Expr=(2*(u(4)*u(3)+u(1)*u(2)))/(1-2*(u(2)^2+u(3)^2))
  y-theta1 : Fcn  Expr=-2*(u(4)*u(2)-u(1)*u(3))
  z-psi1 : Fcn  Expr=(2*(u(2)*u(3)+u(1)*u(4)))/(1-2*(u(4)^2+u(3)^2))
  angle_est : Outport
  wires:
  Gain/1 -> Integrator/1, Quaternion Inverse/1
  Fcn/1 -> Mux1/1
  Fcn3/1 -> Mux1/4
  Mux1/1 -> Gain/1
  Fcn1/1 -> Mux1/2
  Fcn2/1 -> Mux1/3
  Integrator/1 -> Quaternion Normalize/1
  Mux/1 -> Fcn3/1, Fcn2/1, Fcn1/1, Fcn/1
  z-psi1/1 -> Trigonometric Function5/1
  Trigonometric Function4/1 -> Mux2/1
  x-fai1/1 -> Trigonometric Function4/1
  Trigonometric Function3/1 -> Mux2/2
  y-theta1/1 -> Trigonometric Function3/1
  Mux2/1 -> Scope3/1, angle_est/1, Angle Conversion1/1
  Trigonometric Function5/1 -> Mux2/3
  Angle Conversion1/1 -> Scope2/1
  Quaternion Normalize/1 -> Scope4/1, z-psi1/1, y-theta1/1, x-fai1/1, Mux/1
  Demux1/2 -> Trigonometric Function6/1, Trigonometric Function/1
  Demux1/1 -> Trigonometric Function2/1, Trigonometric Function1/1
  Trigonometric Function1/1 -> Divide4/2, Divide5/2, Divide/1
  Demux/2 -> Divide5/1, Divide3/1, Divide/2
  Divide/1 -> Add/1
  Trigonometric Function2/1 -> Divide6/2, Divide3/2, Divide1/2
  Demux/3 -> Divide6/1, Divide4/1, Divide1/1
  Divide1/1 -> Add/2
  Add/1 -> Divide2/1
  Trigonometric Function/1 -> Divide2/2
  Divide2/1 -> Add1/1
  Demux/1 -> Add1/2
  Add1/1 -> Mux3/1
  Divide3/1 -> Add2/1
  Divide4/1 -> Add2/2
  Add2/1 -> Mux3/2
  Divide5/1 -> Add3/1
  Divide6/1 -> Add3/2
  Add3/1 -> Divide7/1
  Trigonometric Function6/1 -> Divide7/2
  Divide7/1 -> Mux3/3
  Mux3/1 -> Integrator1/1
  Integrator1/1 -> Angle Conversion2/1, Demux1/1
  Angle Conversion2/1 -> Scope1/1
  gyro_b/1 -> Demux/1, Mux/2  "omega"

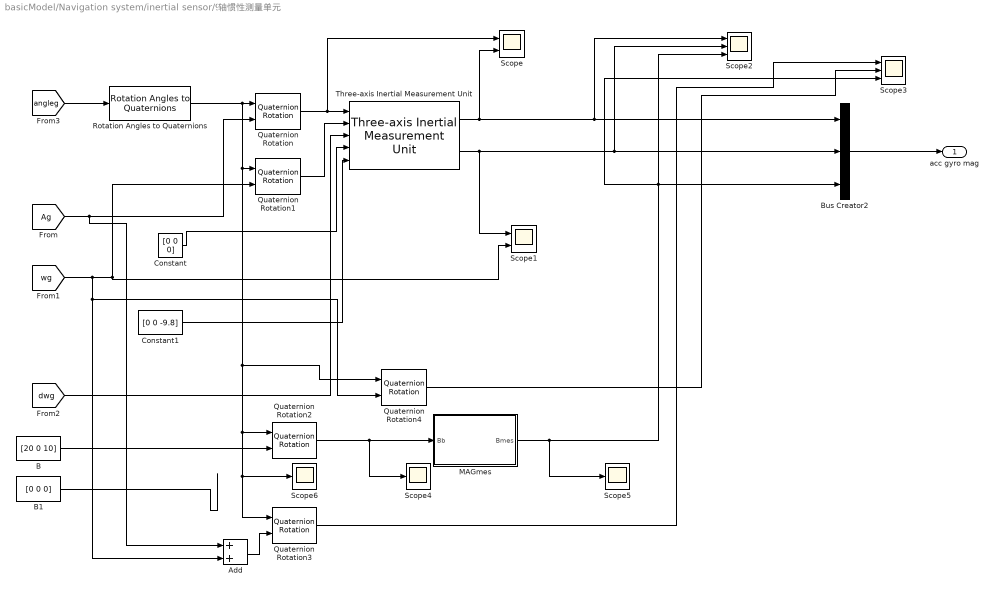
== system basicModel/Navigation system/inertial sensor/9轴惯性测量单元 ==
  Add : Sum
  B : Constant  Value=[20 0 10]
  B1 : Constant  Value=[0 0 0]
  Bus Creator2 : BusCreator  Inputs=3
  Constant : Constant  Value=[0 0 0]
  Constant1 : Constant  Value=[0 0 -9.8]
  MAGmes : Subsystem
  Quaternion Rotation{,1..4} (5 alike) : aerolibutil/Quaternion Rotation
  Rotation Angles to Quaternions : sharedtransform/Rotation Angles to Quaternions  rotationOrder=ZYX
      settings: SourceProductName=Aerospace Blockset  SourceProductBaseCode=AE
  Scope : Scope  NumInputPorts=2
  Scope1 : Scope  NumInputPorts=2
  Scope2 : Scope  NumInputPorts=3
  Scope3 : Scope  NumInputPorts=3
  Scope4 : Scope
  Scope5 : Scope
  Scope6 : Scope
  Three-axis Inertial Measurement Unit : aerolibnav/Three-axis Inertial Measurement Unit  units=Metric (MKS)  imu=[0 0 0]  i_Ts=0.01  dtype_a=off  w_a=190  z_a=0.707  a_sf_cc=[1 0 0; 0 1 0; 0 0 1]  a_bias=[0 0 0]  a_sat="[-inf  -inf  -inf  inf inf inf]"  dtype_g=off  w_g=190  z_g=0.707  g_sf_cc=[1 0 0; 0 1 0; 0 0 1]  g_bias=[0.0001 0.0001 0.0001]  g_sens=[0 0 0]  g_sat="[-inf  -inf  -inf  inf inf inf]"  i_rand=on  i_seeds=[23093 23094 23095 23096 23097 23098]  i_pow=[0.0001 0.0001 0.0001 0.000001 0.000001 0.000001]
  acc gyro mag : Outport
  wires:
  [wg] -> Quaternion Rotation4/2, Add/2, Scope1/2, Quaternion Rotation1/2
  [Ag] -> Add/1, Quaternion Rotation/2
  Rotation Angles to Quaternions/1 -> Quaternion Rotation4/1, Quaternion Rotation2/1, Scope6/1, Quaternion Rotation3/1, Quaternion Rotation1/1, Quaternion Rotation/1
  [dwg] -> Three-axis Inertial Measurement Unit/3
  Constant1/1 -> Three-axis Inertial Measurement Unit/5
  Quaternion Rotation/1 -> Scope/1, Three-axis Inertial Measurement Unit/1
  Constant/1 -> Three-axis Inertial Measurement Unit/4
  Three-axis Inertial Measurement Unit/1 -> Bus Creator2/1, Scope2/1, Scope/2
  Quaternion Rotation1/1 -> Three-axis Inertial Measurement Unit/2
  Bus Creator2/1 -> acc gyro mag/1
  B/1 -> Quaternion Rotation2/2
  Three-axis Inertial Measurement Unit/2 -> Scope1/1, Bus Creator2/2, Scope2/2
  MAGmes/1(Bmes) -> Scope5/1, Scope3/3, Bus Creator2/3, Scope2/3
  Quaternion Rotation2/1 -> Scope4/1, MAGmes/1(Bb)
  [angleg] -> Rotation Angles to Quaternions/1
  Add/1 -> Quaternion Rotation3/2
  Quaternion Rotation3/1 -> Scope3/1
  Quaternion Rotation4/1 -> Scope3/2
  B1/1 -> ?

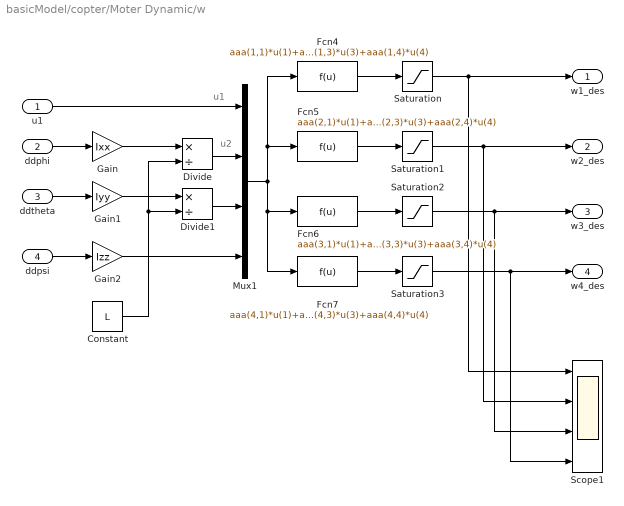
== system basicModel/copter/Moter Dynamic/w ==
  note: u2
  note: u1
  u1 : Inport
  ddphi : Inport  Port=2
  ddtheta : Inport  Port=3
  ddpsi : Inport  Port=4
  Constant : Constant  Value=L
  Divide : Product  Inputs=*/
  Divide1 : Product  Inputs=*/
  Fcn4 : Fcn  Expr=aaa(1,1)*u(1)+aaa(1,2)*u(2)+aaa(1,3)*u(3)+aaa(1,4)*u(4)
  Fcn5 : Fcn  Expr=aaa(2,1)*u(1)+aaa(2,2)*u(2)+aaa(2,3)*u(3)+aaa(2,4)*u(4)
  Fcn6 : Fcn  Expr=aaa(3,1)*u(1)+aaa(3,2)*u(2)+aaa(3,3)*u(3)+aaa(3,4)*u(4)
  Fcn7 : Fcn  Expr=aaa(4,1)*u(1)+aaa(4,2)*u(2)+aaa(4,3)*u(3)+aaa(4,4)*u(4)
  Gain : Gain  Gain=Ixx
  Gain1 : Gain  Gain=Iyy
  Gain2 : Gain  Gain=Izz
  Mux1 : Mux
  Saturation{,1..3} (4 alike) : Saturate  UpperLimit=(6000*2*pi/60)^2  LowerLimit=0
  Scope1 : Scope  NumInputPorts=4
  w1_des : Outport
  w2_des : Outport  Port=2
  w3_des : Outport  Port=3
  w4_des : Outport  Port=4
  wires:
  u1/1 -> Mux1/1
  ddphi/1 -> Gain/1
  ddpsi/1 -> Gain2/1
  ddtheta/1 -> Gain1/1
  Mux1/1 -> Fcn5/1, Fcn4/1, Fcn7/1, Fcn6/1
  Fcn4/1 -> Saturation/1
  Fcn6/1 -> Saturation2/1
  Fcn7/1 -> Saturation3/1
  Saturation/1 -> Scope1/1, w1_des/1
  Saturation1/1 -> Scope1/2, w2_des/1
  Saturation2/1 -> Scope1/3, w3_des/1
  Saturation3/1 -> Scope1/4, w4_des/1
  Divide/1 -> Mux1/2
  Gain/1 -> Divide/1
  Constant/1 -> Divide1/2, Divide/2
  Divide1/1 -> Mux1/3
  Gain2/1 -> Mux1/4
  Gain1/1 -> Divide1/1
  Fcn5/1 -> Saturation1/1

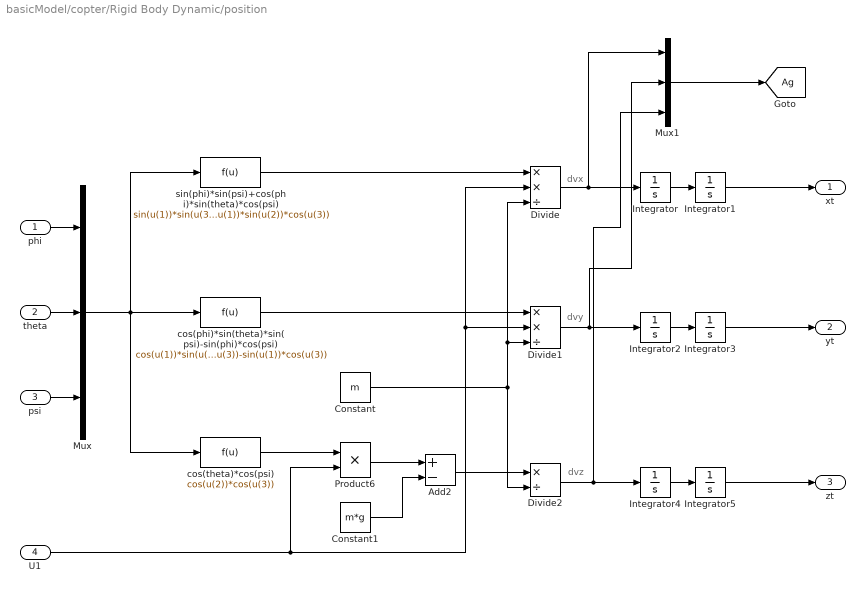
== system basicModel/copter/Rigid Body Dynamic/position ==
  note: dvz
  note: dvy
  note: dvx
  phi : Inport
  theta : Inport  Port=2
  psi : Inport  Port=3
  U1 : Inport  Port=4
  Add2 : Sum  Inputs=+-
  Constant : Constant  Value=m
  Constant1 : Constant  Value=m*g
  Divide : Product  Inputs=**/
  Divide1 : Product  Inputs=**/
  Divide2 : Product  Inputs=*/
  Integrator{,1..5} (6 alike) : Integrator
  Mux : Mux  Inputs=3
  Mux1 : Mux  Inputs=3
  Product6 : Product
  cos(phi)*sin(theta)*sin(psi)-sin(phi)*cos(psi) : Fcn  Expr=cos(u(1))*sin(u(2))*sin(u(3))-sin(u(1))*cos(u(3))
  cos(theta)*cos(psi) : Fcn  Expr=cos(u(2))*cos(u(3))
  sin(phi)*sin(psi)+cos(phi)*sin(theta)*cos(psi) : Fcn  Expr=sin(u(1))*sin(u(3))+cos(u(1))*sin(u(2))*cos(u(3))
  xt : Outport
  yt : Outport  Port=2
  zt : Outport  Port=3
  tag scope: Ag=global
  wires:
  phi/1 -> Mux/1
  theta/1 -> Mux/2
  Integrator/1 -> Integrator1/1
  Integrator2/1 -> Integrator3/1
  Integrator4/1 -> Integrator5/1
  Integrator5/1 -> zt/1
  Integrator3/1 -> yt/1
  Integrator1/1 -> xt/1
  Divide/1 -> Mux1/1, Integrator/1
  U1/1 -> Product6/2, Divide/2, Divide1/2
  Divide1/1 -> Mux1/2, Integrator2/1
  Divide2/1 -> Mux1/3, Integrator4/1
  Constant1/1 -> Add2/2
  Product6/1 -> Add2/1
  Constant/1 -> Divide2/2, Divide/3, Divide1/3
  cos(phi)*sin(theta)*sin(psi)-sin(phi)*cos(psi)/1 -> Divide1/1
  Add2/1 -> Divide2/1
  psi/1 -> Mux/3
  Mux/1 -> sin(phi)*sin(psi)+cos(phi)*sin(theta)*cos(psi)/1, cos(theta)*cos(psi)/1, cos(phi)*sin(theta)*sin(psi)-sin(phi)*cos(psi)/1
  sin(phi)*sin(psi)+cos(phi)*sin(theta)*cos(psi)/1 -> Divide/1
  cos(theta)*cos(psi)/1 -> Product6/1
  Mux1/1 -> [Ag]

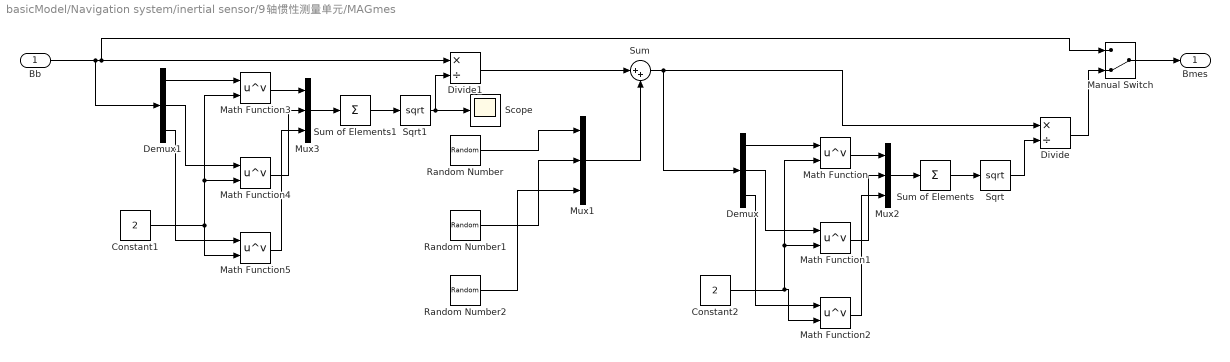
== system basicModel/Navigation system/inertial sensor/9轴惯性测量单元/MAGmes ==
  Bb : Inport
  Constant1 : Constant  Value=2
  Constant2 : Constant  Value=2
  Demux : Demux  Outputs=3
  Demux1 : Demux  Outputs=3
  Divide : Product  Inputs=*/
  Divide1 : Product  Inputs=*/
  Manual Switch : ManualSwitch  CurrentSetting=0
  Math Function{,1..5} (6 alike) : Math  Operator=pow  SaturateOnIntegerOverflow=on
  Mux1 : Mux  Inputs=3
  Mux2 : Mux  Inputs=3
  Mux3 : Mux  Inputs=3
  Random Number : RandomNumber  Variance=0.0001  Seed=22  SampleTime=0.01
  Random Number1 : RandomNumber  Variance=0.0001  Seed=23  SampleTime=0.01
  Random Number2 : RandomNumber  Variance=0.0001  Seed=24  SampleTime=0.01
  Scope : Scope
  Sqrt : Sqrt  SaturateOnIntegerOverflow=on
  Sqrt1 : Sqrt  SaturateOnIntegerOverflow=on
  Sum : Sum  Inputs=|++
  Sum of Elements : Sum  Inputs=+
  Sum of Elements1 : Sum  Inputs=+
  Bmes : Outport
  wires:
  Divide/1 -> Manual Switch/2
  Mux2/1 -> Sum of Elements/1
  Sum of Elements/1 -> Sqrt/1
  Sqrt/1 -> Divide/2
  Math Function2/1 -> Mux2/3
  Math Function/1 -> Mux2/1
  Constant2/1 -> Math Function2/2, Math Function1/2, Math Function/2
  Demux/3 -> Math Function2/1
  Math Function1/1 -> Mux2/2
  Random Number1/1 -> Mux1/2
  Random Number2/1 -> Mux1/3
  Sum/1 -> Demux/1, Divide/1
  Demux/2 -> Math Function1/1
  Random Number/1 -> Mux1/1
  Demux/1 -> Math Function/1
  Divide1/1 -> Sum/1
  Mux3/1 -> Sum of Elements1/1
  Sum of Elements1/1 -> Sqrt1/1
  Sqrt1/1 -> Scope/1, Divide1/2
  Math Function5/1 -> Mux3/3
  Math Function3/1 -> Mux3/1
  Constant1/1 -> Math Function4/2, Math Function3/2, Math Function5/2
  Demux1/3 -> Math Function5/1
  Math Function4/1 -> Mux3/2
  Bb/1 -> Demux1/1, Manual Switch/1, Divide1/1
  Demux1/2 -> Math Function4/1
  Demux1/1 -> Math Function3/1
  Manual Switch/1 -> Bmes/1
  Mux1/1 -> Sum/2

== matlab function basicModel/Navigation system/Attitude estimate/地磁传感器直接解算偏航角/MATLAB Function ==
  data: u input; y output
function y = fcn(u)
fai=u(1);
theta=u(2);
psi=u(3);
psi=0;
bx=u(4);
by=u(5);
bz=u(6);
% f = (cos(psi)*cos(theta)*(cos(psi)*sin(fai) - cos(fai)*sin(psi)*sin(theta)) + cos(theta)*sin(psi)*(sin(fai)*sin(psi) + cos(fai)*cos(psi)*sin(theta)))*(by*(sin(fai)*sin(psi) + cos(fai)*cos(psi)*sin(theta)) + bz*(cos(fai)*sin(psi) - cos(psi)*sin(fai)*sin(theta))) - bx*(sin(fai)*sin(psi) + cos(fai)*cos(psi)*sin(theta))*((sin(fai)*sin(psi) + cos(fai)*cos(psi)*sin(theta))*(cos(fai)*cos(psi) + sin(fai)*sin(psi)*sin(theta)) - (cos(fai)*sin(psi) - cos(psi)*sin(fai)*sin(theta))*(cos(psi)*sin(fai) - cos(fai)*sin(psi)*sin(theta))) + bz*cos(psi)*cos(theta)*((sin(fai)*sin(psi) + cos(fai)*cos(psi)*sin(theta))*(cos(fai)*cos(psi) + sin(fai)*sin(psi)*sin(theta)) - (cos(fai)*sin(psi) - cos(psi)*sin(fai)*sin(theta))*(cos(psi)*sin(fai) - cos(fai)*sin(psi)*sin(theta)));
% % df_psi=(cos(psi)*cos(theta)*(cos(psi)*sin(fai) - cos(fai)*sin(psi)*sin(theta)) + cos(theta)*sin(psi)*(sin(fai)*sin(psi) + cos(fai)*cos(psi)*sin(theta)))*(by*(cos(psi)*sin(fai) - cos(fai)*sin(psi)*sin(theta)) + bz*(cos(fai)*cos(psi) + sin(fai)*sin(psi)*sin(theta))) - bx*(cos(psi)*sin(fai) - cos(fai)*sin(psi)*sin(theta))*((sin(fai)*sin(psi) + cos(fai)*cos(psi)*sin(theta))*(cos(fai)*cos(psi) + sin(fai)*sin(psi)*sin(theta)) - (cos(fai)*sin(psi) - cos(psi)*sin(fai)*sin(theta))*(cos(psi)*sin(fai) - cos(fai)*sin(psi)*sin(theta))) - bz*cos(theta)*sin(psi)*((sin(fai)*sin(psi) + cos(fai)*cos(psi)*sin(theta))*(cos(fai)*cos(psi) + sin(fai)*sin(psi)*sin(theta)) - (cos(fai)*sin(psi) - cos(psi)*sin(fai)*sin(theta))*(cos(psi)*sin(fai) - cos(fai)*sin(psi)*sin(theta)));
% N =1000;
% x0=0;
% x1=f;
% E=1.0e-6;%f=x*x*x+4*x*x-10=0,f1为f=x*x*x+4*x*x-10的一阶导
% k=1;
% while(norm(x1-x0)>=E&&k<N)
% 	x0=x1;
% 	f=(cos(psi)*cos(theta)*(cos(psi)*sin(fai) - cos(fai)*sin(psi)*sin(theta)) + cos(theta)*sin(psi)*(sin(fai)*sin(psi) + cos(fai)*cos(psi)*sin(theta)))*(by*(sin(fai)*sin(psi) + cos(fai)*cos(psi)*sin(theta)) + bz*(cos(fai)*sin(psi) - cos(psi)*sin(fai)*sin(theta))) - bx*(sin(fai)*sin(psi) + cos(fai)*cos(psi)*sin(theta))*((sin(fai)*sin(psi) + cos(fai)*cos(psi)*sin(theta))*(cos(fai)*cos(psi) + sin(fai)*sin(psi)*sin(theta)) - (cos(fai)*sin(psi) - cos(psi)*sin(fai)*sin(theta))*(cos(psi)*sin(fai) - cos(fai)*sin(psi)*sin(theta))) + bz*cos(psi)*cos(theta)*((sin(fai)*sin(psi) + cos(fai)*cos(psi)*sin(theta))*(cos(fai)*cos(psi) + sin(fai)*sin(psi)*sin(theta)) - (cos(fai)*sin(psi) - cos(psi)*sin(fai)*sin(theta))*(cos(psi)*sin(fai) - cos(fai)*sin(psi)*sin(theta)));
% 	f1=(cos(psi)*cos(theta)*(cos(psi)*sin(fai) - cos(fai)*sin(psi)*sin(theta)) + cos(theta)*sin(psi)*(sin(fai)*sin(psi) + cos(fai)*cos(psi)*sin(theta)))*(by*(cos(psi)*sin(fai) - cos(fai)*sin(psi)*sin(theta)) + bz*(cos(fai)*cos(psi) + sin(fai)*sin(psi)*sin(theta))) - bx*(cos(psi)*sin(fai) - cos(fai)*sin(psi)*sin(theta))*((sin(fai)*sin(psi) + cos(fai)*cos(psi)*sin(theta))*(cos(fai)*cos(psi) + sin(fai)*sin(psi)*sin(theta)) - (cos(fai)*sin(psi) - cos(psi)*sin(fai)*sin(theta))*(cos(psi)*sin(fai) - cos(fai)*sin(psi)*sin(theta))) - bz*cos(theta)*sin(psi)*((sin(fai)*sin(psi) + cos(fai)*cos(psi)*sin(theta))*(cos(fai)*cos(psi) + sin(fai)*sin(psi)*sin(theta)) - (cos(fai)*sin(psi) - cos(psi)*sin(fai)*sin(theta))*(cos(psi)*sin(fai) - cos(fai)*sin(psi)*sin(theta)));
% 	if(f1~=0)
% 		x1=x0-f/f1;
% 	end
% 	k=k+1;
% end
% if x1>2*pi
% 	x1 = mod(x1,2*pi);
% end
% if x1<0
% 	x1 = mod(x1,-2*pi);
% 	x1 = x1+2*pi;
% end
% % if x1 > pi
% % 	x1 =-(pi-( x1-pi));
% % end
% y = x1;
A = bx*cos(theta)+by*sin(fai)*sin(theta)+bz*cos(fai)*sin(theta);
B = by*cos(fai)-bz*sin(fai);
psi = -atan(B/A);

% psi = mod(psi,2*pi);

y = psi;
